simulink model "bicycle_func"  (R2020a)
settings: Solver=VariableStepAuto  StartTime=0.0  StopTime=10.0  RelTol=1e-3
settings Model: Creator=exorcist  LastModifiedBy=exorcist

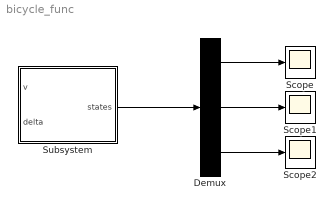
== system bicycle_func ==
  Demux : Demux  Outputs=3
  Scope : Scope
  Scope1 : Scope
  Scope2 : Scope
  Subsystem : Subsystem
  wires:
  Subsystem/1(states) -> Demux/1
  Demux/1 -> Scope/1
  Demux/2 -> Scope1/1
  Demux/3 -> Scope2/1

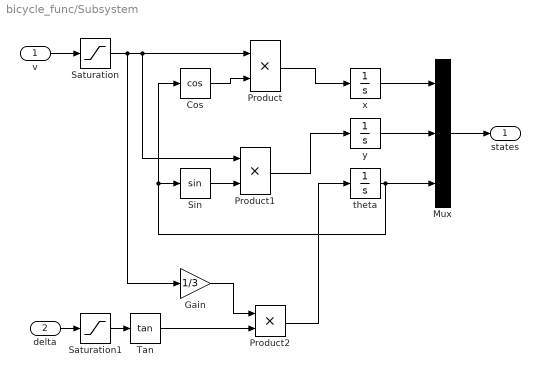
== system bicycle_func/Subsystem ==
  v : Inport
  delta : Inport  Port=2
  Cos : Trigonometry  Operator=cos
  Gain : Gain  Gain=1/3
  Mux : Mux  Inputs=3
  Product : Product
  Product1 : Product
  Product2 : Product
  Saturation : Saturate  UpperLimit=12  LowerLimit=0
  Saturation1 : Saturate  UpperLimit=pi/4  LowerLimit=-pi/4
  Sin : Trigonometry
  Tan : Trigonometry  Operator=tan
  theta : Integrator
  x : Integrator
  y : Integrator  InitialCondition=-3
  states : Outport
  wires:
  x/1 -> Mux/1
  y/1 -> Mux/2
  theta/1 -> Cos/1, Sin/1, Mux/3
  Mux/1 -> states/1
  Cos/1 -> Product/2
  Product/1 -> x/1
  Product1/1 -> y/1
  Sin/1 -> Product1/2
  Tan/1 -> Product2/2
  Gain/1 -> Product2/1
  Product2/1 -> theta/1
  v/1 -> Saturation/1
  Saturation/1 -> Gain/1, Product1/1, Product/1
  delta/1 -> Saturation1/1
  Saturation1/1 -> Tan/1
